simulink model "Motor_Dynamics_practice2_final_2024b"  (R2024b)
settings: Solver=VariableStepAuto  StartTime=0.0  StopTime=1  RelTol=1e-3
InitFcn:
  | %% environmental parameter
  | 
  | g = 9.81;                       %[m/ss]
  | 
  | %% Vehicle parameter
  | 
  | mass = 1.5;                     %[kg]
  | Arm_Length = 0.225;             %[m]
  | 
  | %% Motor parameter
  | 
  | rad2rpm = 60 / (2 * pi);
  | 
  | rpm2rad = 1 / rad2rpm;
  | 
  | Friction_Coef = 0.0001;         %[N m /s]
  | 
  | Inertia = 2.8e-05;              %[kg m^2]
  | 
  | Resistance = 0.1170;            %[ohm]
  | 
  | K_Torque = 1 / (rpm2rad * 960); %[N m/A]
  | 
  | K_Emf = K_Torque;               %[V s/rad]
  | 
  | Tau = (Inertia * Resistance) / (Resistance * Friction_Coef + K_Torque + K_Emf);
  | 
  | ks = K_Torque / (Resistance * Friction_Coef + K_Torque * K_Emf);
  | 
  | Thrust_Coef = 1.1768e-05;
  | 
  | Drag_Coef = 1.8542e-07;
  | 
  | Hovering_Motor_Speed = sqrt(mass * g / (4 * Thrust_Coef));
settings Model: Creator=user  LastModifiedBy=user

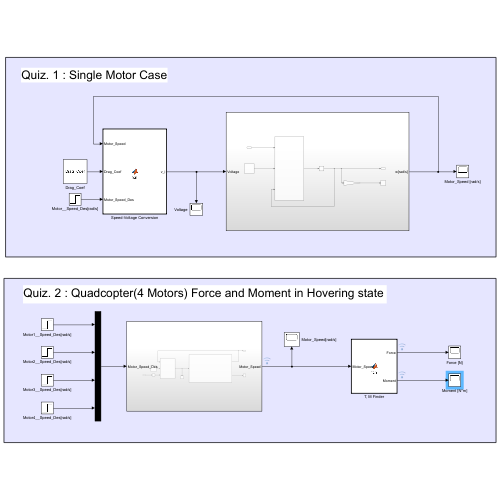
[thumbnail: Simulink's stored preview of the top-level diagram]
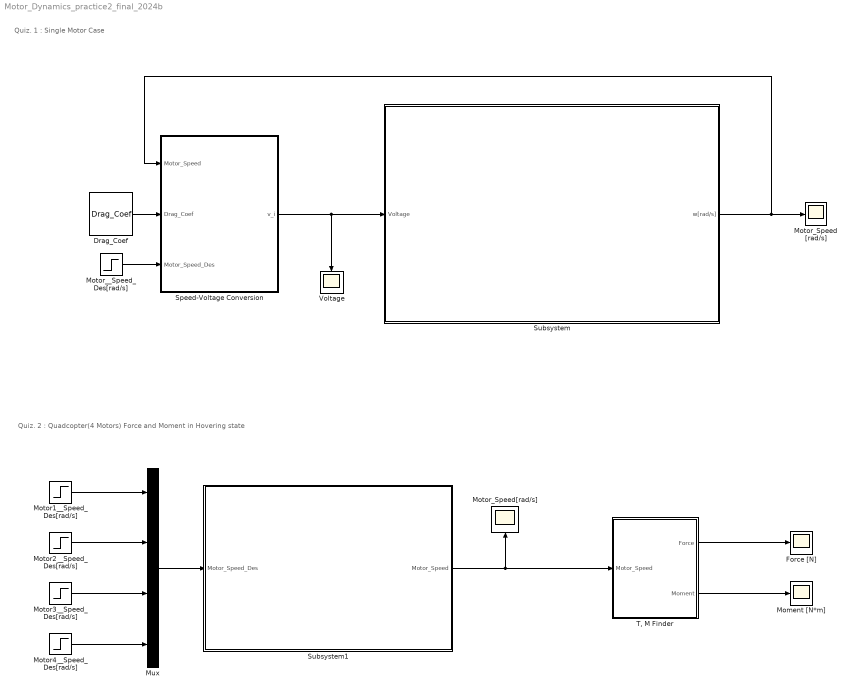
== system Motor_Dynamics_practice2_final_2024b ==
  note: Quiz. 2 : Quadcopter(4 Motors) Force and Moment in Hovering state
  note: Quiz. 1 : Single Motor Case
  Drag_Coef : Constant  Value=Drag_Coef
  Force [N] : Scope
  Moment [N*m] : Scope
  Motor1__Speed_Des[rad/s] : Step  Time=0  After=Hovering_Motor_Speed  SampleTime=0
  Motor2__Speed_Des[rad/s] : Step  Time=0  After=Hovering_Motor_Speed  SampleTime=0
  Motor3__Speed_Des[rad/s] : Step  Time=0  After=Hovering_Motor_Speed  SampleTime=0
  Motor4__Speed_Des[rad/s] : Step  Time=0  After=Hovering_Motor_Speed  SampleTime=0
  Motor_Speed [rad/s] : Scope
  Motor_Speed[rad/s] : Scope
  Motor__Speed_Des[rad/s] : Step  Time=0  After=Hovering_Motor_Speed  SampleTime=0
  Mux : Mux
  Speed-Voltage Conversion : MATLAB Function  TreatAsAtomicUnit=on
  Subsystem : Subsystem
  Subsystem1 : Subsystem
  "T, M Finder" : MATLAB Function  TreatAsAtomicUnit=on
  Voltage : Scope
  wires:
  Motor1__Speed_Des[rad/s]/1 -> Mux/1
  Motor2__Speed_Des[rad/s]/1 -> Mux/2
  Motor3__Speed_Des[rad/s]/1 -> Mux/3
  Motor4__Speed_Des[rad/s]/1 -> Mux/4
  Mux/1 -> Subsystem1/1(Motor_Speed_Des)
  Subsystem1/1(Motor_Speed) -> "T, M Finder"/1(Motor_Speed), Motor_Speed[rad/s]/1
  "T, M Finder"/2(Moment) -> Moment [N*m]/1
  "T, M Finder"/1(Force) -> Force [N]/1
  Motor__Speed_Des[rad/s]/1 -> Speed-Voltage Conversion/3(Motor_Speed_Des)
  Speed-Voltage Conversion/1(v_i) -> Voltage/1, Subsystem/1(Voltage)
  Drag_Coef/1 -> Speed-Voltage Conversion/2(Drag_Coef)
  Subsystem/1(w[rad/s]) -> Speed-Voltage Conversion/1(Motor_Speed), Motor_Speed [rad/s]/1

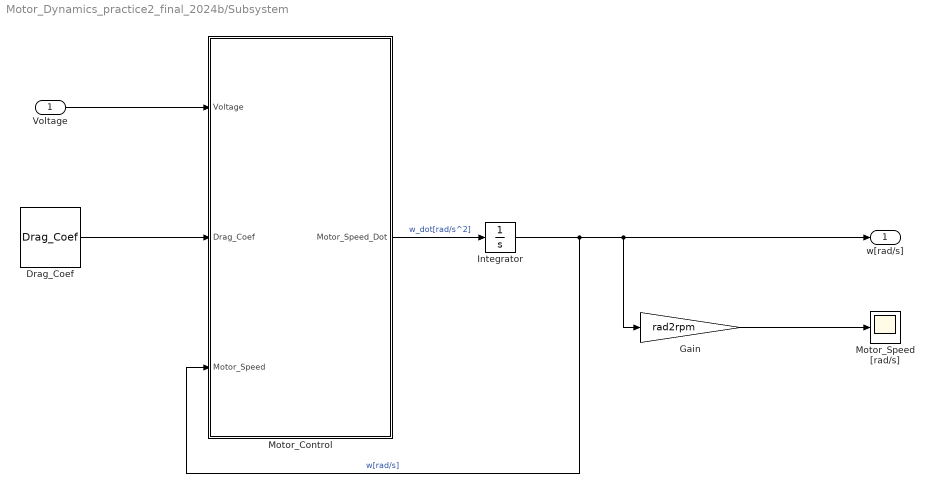
== system Motor_Dynamics_practice2_final_2024b/Subsystem ==
  Voltage : Inport
  Drag_Coef : Constant  Value=Drag_Coef
  Gain : Gain  Gain=rad2rpm
  Integrator : Integrator
  Motor_Control : MATLAB Function  TreatAsAtomicUnit=on
  Motor_Speed [rad/s] : Scope
  w[rad/s] : Outport
  wires:
  Motor_Control/1(Motor_Speed_Dot) -> Integrator/1  "w_dot[rad/s^2]"
  Integrator/1 -> w[rad/s]/1, Gain/1, Motor_Control/3(Motor_Speed)  "w[rad/s]"
  Gain/1 -> Motor_Speed [rad/s]/1
  Voltage/1 -> Motor_Control/1(Voltage)
  Drag_Coef/1 -> Motor_Control/2(Drag_Coef)

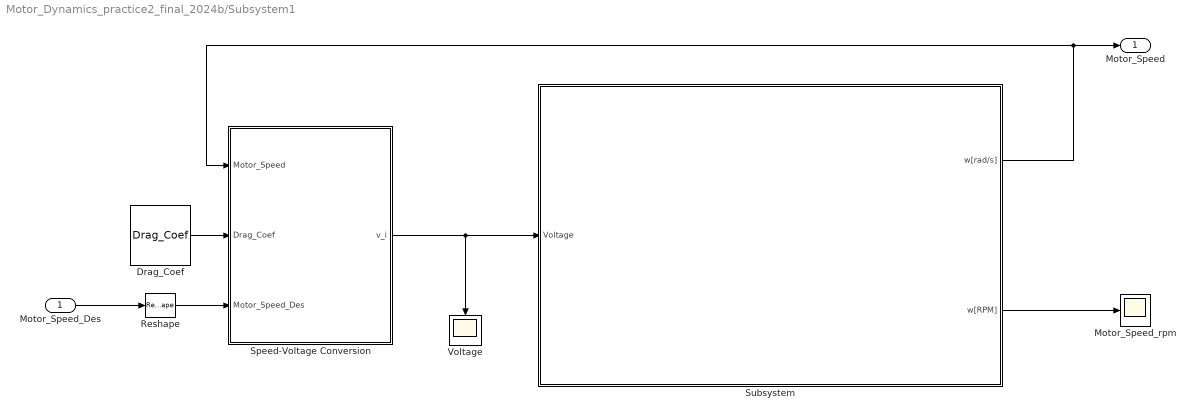
== system Motor_Dynamics_practice2_final_2024b/Subsystem1 ==
  Motor_Speed_Des : Inport
  Drag_Coef : Constant  Value=Drag_Coef
  Motor_Speed_rpm : Scope
  Reshape : Reshape  OutputDimensionality=Column vector (2-D)
  Speed-Voltage Conversion : MATLAB Function  TreatAsAtomicUnit=on
  Subsystem : Subsystem
  Voltage : Scope
  Motor_Speed : Outport
  wires:
  Speed-Voltage Conversion/1(v_i) -> Voltage/1, Subsystem/1(Voltage)
  Drag_Coef/1 -> Speed-Voltage Conversion/2(Drag_Coef)
  Subsystem/1(w[rad/s]) -> Motor_Speed/1, Speed-Voltage Conversion/1(Motor_Speed)
  Subsystem/2(w[RPM]) -> Motor_Speed_rpm/1
  Motor_Speed_Des/1 -> Reshape/1
  Reshape/1 -> Speed-Voltage Conversion/3(Motor_Speed_Des)

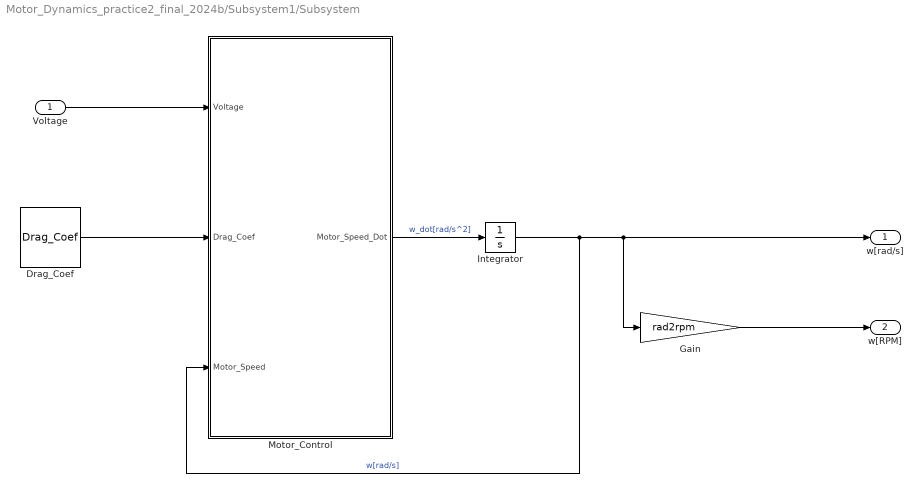
== system Motor_Dynamics_practice2_final_2024b/Subsystem1/Subsystem ==
  Voltage : Inport
  Drag_Coef : Constant  Value=Drag_Coef
  Gain : Gain  Gain=rad2rpm
  Integrator : Integrator  InitialCondition=[0 0 0 0]'
  Motor_Control : MATLAB Function  TreatAsAtomicUnit=on
  w[rad/s] : Outport
  w[RPM] : Outport  Port=2
  wires:
  Motor_Control/1(Motor_Speed_Dot) -> Integrator/1  "w_dot[rad/s^2]"
  Integrator/1 -> w[rad/s]/1, Gain/1, Motor_Control/3(Motor_Speed)  "w[rad/s]"
  Gain/1 -> w[RPM]/1
  Voltage/1 -> Motor_Control/1(Voltage)
  Drag_Coef/1 -> Motor_Control/2(Drag_Coef)

== matlab function Motor_Dynamics_practice2_final_2024b/Subsystem1/Speed-Voltage Conversion ==
  data: Motor_Speed input; Drag_Coef input; Motor_Speed_Des input; v_i output
function v_i = fcn(Motor_Speed, Drag_Coef, Motor_Speed_Des)

rad2rpm = 60 / (2 * pi);

rpm2rad = 1 / rad2rpm;

Resistance = 0.1170;            %[ohm]

K_Torque = 1 / (rpm2rad * 960); %[N m/A]

K_Emf = K_Torque;               %[V s/rad]


v_i = K_Emf .* Motor_Speed_Des + Resistance/K_Torque * Drag_Coef .* Motor_Speed.^2;


end

== matlab function Motor_Dynamics_practice2_final_2024b/Subsystem1/Subsystem/Motor_Control ==
  data: Voltage input; Drag_Coef input; Motor_Speed_Dot output; Motor_Speed input
function Motor_Speed_Dot = fcn(Voltage, Drag_Coef, Motor_Speed)

rad2rpm = 60 / (2 * pi);

rpm2rad = 1 / rad2rpm;

Inertia = 2.8e-05;              %[kg m^2]

Resistance = 0.1170;            %[ohm]

K_Torque = 1 / (rpm2rad * 960); %[N m/A]

K_Emf = K_Torque;               %[V s/rad]

V_Emf = K_Emf .* Motor_Speed; %[Voltage]

Current = (Voltage - V_Emf) / Resistance; %[A]

Motor_Speed_Dot = (K_Torque * Current - Drag_Coef * Motor_Speed.^2)/ Inertia; %[rad/s^2]

end

== matlab function Motor_Dynamics_practice2_final_2024b/T, M Finder ==
  data: Motor_Speed input; Force output; Moment output
function [Force, Moment] = fcn(Motor_Speed)

Thrust_Coef = 1.1768e-05;

Drag_Coef = 1.8542e-07;

Arm_Length = 0.225;             %[m]


Force = [0;
         0;
         -Thrust_Coef * sum(Motor_Speed.^2)];


Drag = Drag_Coef * Motor_Speed.^2; %4x1 matrix, [d] .* [w^2]


Moment = [Arm_Length * Thrust_Coef * (Motor_Speed(4)^2 - Motor_Speed(2)^2);
          Arm_Length * Thrust_Coef * (Motor_Speed(1)^2 - Motor_Speed(3)^2);
          -Drag(1) + Drag(2) - Drag(3) + Drag(4)];

== matlab function Motor_Dynamics_practice2_final_2024b/Speed-Voltage Conversion ==
  data: Motor_Speed input; Drag_Coef input; Motor_Speed_Des input; v_i output
function v_i = fcn(Motor_Speed, Drag_Coef, Motor_Speed_Des)

rad2rpm = 60 / (2 * pi);

rpm2rad = 1 / rad2rpm;

Resistance = 0.1170;            %[ohm]

K_Torque = 1 / (rpm2rad * 960); %[N m/A]

K_Emf = K_Torque;               %[V s/rad]


v_i = K_Emf * Motor_Speed_Des + Resistance/K_Torque * Drag_Coef * Motor_Speed^2;


end

== matlab function Motor_Dynamics_practice2_final_2024b/Subsystem/Motor_Control ==
  data: Voltage input; Drag_Coef input; Motor_Speed_Dot output; Motor_Speed input
function Motor_Speed_Dot = fcn(Voltage, Drag_Coef, Motor_Speed)

rad2rpm = 60 / (2 * pi);

rpm2rad = 1 / rad2rpm;

Inertia = 2.8e-05;              %[kg m^2]

Resistance = 0.1170;            %[ohm]

K_Torque = 1 / (rpm2rad * 960); %[N m/A]

K_Emf = K_Torque;               %[V s/rad]

V_Emf = K_Emf * Motor_Speed; %[Voltage]

Current = (Voltage - V_Emf) / Resistance; %[A]

Motor_Speed_Dot = (K_Torque * Current - Drag_Coef * Motor_Speed^2)/ Inertia; %[rad/s^2]

end
